simulink subsystem "receive_blocker"  (R2021b)
settings: Solver=VariableStepAuto  StartTime=0.0  StopTime=10.0  RelTol=1e-3
undefined symbols (not defined in the file): antenna_num, sample_bitwidth
settings Model: Creator=torha  LastModifiedBy=torha
settings SolverCC: AlgebraicLoopSolver=TrustRegion
settings DebuggingCC: SFMachineParentedDataDiag=warning

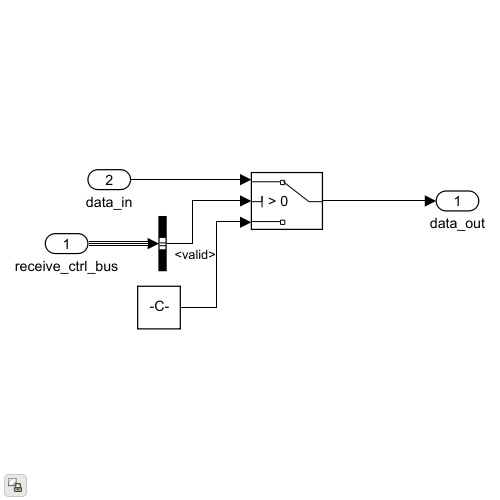
[thumbnail: Simulink's stored preview of the top-level diagram]
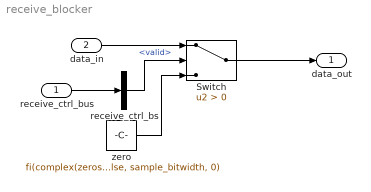
== system receive_blocker ==
  receive_ctrl_bus : Inport
  data_in : Inport  Port=2
  Switch : Switch  Criteria=u2 > Threshold
  receive_ctrl_bs : BusSelector  OutputSignals=valid
  zero : Constant  Value=fi(complex(zeros(1, antenna_num)), false, sample_bitwidth, 0)
  data_out : Outport
  wires:
  receive_ctrl_bs/1 -> Switch/2  "<valid>"
  receive_ctrl_bus/1 -> receive_ctrl_bs/1
  zero/1 -> Switch/3
  Switch/1 -> data_out/1
  data_in/1 -> Switch/1
